simulink model "LSSB"  (R2013b)
settings: Solver=ode45  StartTime=0.0  StopTime=10.0  RelTol=1e-3
undefined symbols (not defined in the file): fdesignblkfcn, gcbh
libraries: dspsrcs4 x1
settings Model: Creator=Nouri  LastModifiedBy=Nouri

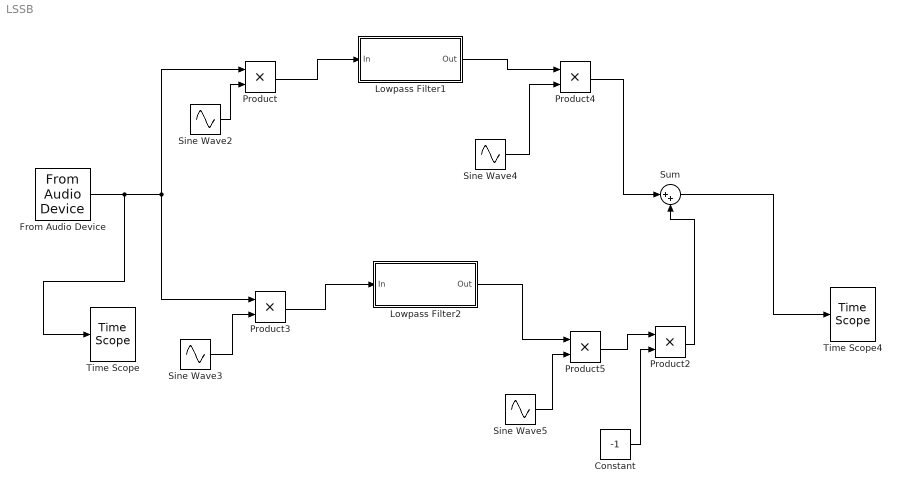
== system LSSB ==
  Constant : Constant  Value=-1
  From Audio Device : dspsrcs4/From Audio Device  deviceName=Default  numChannels=1  sampleRate=44000  deviceDatatype=Determine from output data type  autoBufferSize=on  bufferSize=4096  queueDuration=5  frameSize=1  outputDatatype=single  defaultInputChannelMapping=on  inputChannelMapping=1:2
  Lowpass Filter1 : Subsystem  DialogController=fdesignblkfcn  InitFcn=fdesignblkfcn(gcbh, {'InitFcn'});  mask(Lowpass Filter){}
      mask help: Design a lowpass filter
      settings: CopyFcn=fdesignblkfcn(gcbh, {'CopyFcn'});
      mask Help: helpview(mapfilelocation('dsp'), 'dsplowpassfilter');
      mask Display: disp('Lowpass')
  Lowpass Filter2 : Subsystem  DialogController=fdesignblkfcn  InitFcn=fdesignblkfcn(gcbh, {'InitFcn'});  mask(Lowpass Filter){}
      mask help: Design a lowpass filter
      settings: CopyFcn=fdesignblkfcn(gcbh, {'CopyFcn'});
      mask Help: helpview(mapfilelocation('dsp'), 'dsplowpassfilter');
      mask Display: disp('Lowpass')
  Product{,2..5} (5 alike) : Product
  Sine Wave2 : Sin  Amplitude=5  Frequency=22000  Phase=pi/2  SampleTime=0
  Sine Wave3 : Sin  Amplitude=5  Frequency=22000  SampleTime=0
  Sine Wave4 : Sin  Amplitude=5  Frequency=66000  Phase=pi/2  SampleTime=0
  Sine Wave5 : Sin  Amplitude=5  Frequency=66000  SampleTime=0
  Sum : Sum  Inputs=|++
  Time Scope : TimeScope  DefaultConfigurationName=spbscopes.TimeScopeBlockCfg
      settings: CopyFcn=scopeextensions.ScopeBlock.onCoreBlockCopy(gcbh);  DeleteFcn=scopeextensions.ScopeBlock.callback(gcbh, 'onBlockDelete');  PreSaveFcn=scopeextensions.ScopeBlock.callback(gcbh, 'onModelSave');  NameChangeFcn=scopeextensions.ScopeBlock.callback(gcbh, 'onBlockRename');  DestroyFcn=scopeextensions.ScopeBlock.onBlockDestroy(gcbh)  CloseFcn=scopeextensions.ScopeBlock.callback(gcbh, 'onBlockClose');  PreDeleteFcn=scopeextensions.ScopeBlock.callback(gcbh, 'onBlockPreDelete');
  Time Scope4 : TimeScope  DefaultConfigurationName=spbscopes.TimeScopeBlockCfg
      settings: CopyFcn=scopeextensions.ScopeBlock.onCoreBlockCopy(gcbh);  DeleteFcn=scopeextensions.ScopeBlock.callback(gcbh, 'onBlockDelete');  PreSaveFcn=scopeextensions.ScopeBlock.callback(gcbh, 'onModelSave');  NameChangeFcn=scopeextensions.ScopeBlock.callback(gcbh, 'onBlockRename');  DestroyFcn=scopeextensions.ScopeBlock.onBlockDestroy(gcbh)  CloseFcn=scopeextensions.ScopeBlock.callback(gcbh, 'onBlockClose');  PreDeleteFcn=scopeextensions.ScopeBlock.callback(gcbh, 'onBlockPreDelete');
  wires:
  Sine Wave2/1 -> Product/2
  From Audio Device/1 -> Product/1, Product3/1, Time Scope/1
  Sine Wave3/1 -> Product3/2
  Product/1 -> Lowpass Filter1/1(In)
  Product3/1 -> Lowpass Filter2/1(In)
  Lowpass Filter2/1(Out) -> Product5/1
  Lowpass Filter1/1(Out) -> Product4/1
  Sine Wave4/1 -> Product4/2
  Sine Wave5/1 -> Product5/2
  Product4/1 -> Sum/1
  Sum/1 -> Time Scope4/1
  Product5/1 -> Product2/1
  Constant/1 -> Product2/2
  Product2/1 -> Sum/2

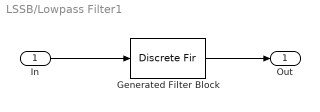
== system LSSB/Lowpass Filter1 ==
  In : Inport
  Generated Filter Block : DiscreteFir  Tag=BlockMethodSubSystem  Coefficients=[-0.0034436495845580231 -0.0059164791571934081 0.0074434606687912869 0.054740018373940491 0.13478679515848707 0.21479383660135923 0.24873045448052369 0.21479383660135923 0.13478679515848707 0.054740018373940491 0.0074434606687912869 -0.0059164791571934081 -0.0034436495845580231]
  Out : Outport
  wires:
  In/1 -> Generated Filter Block/1
  Generated Filter Block/1 -> Out/1

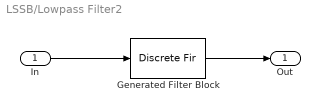
== system LSSB/Lowpass Filter2 ==
  In : Inport
  Generated Filter Block : DiscreteFir  Tag=BlockMethodSubSystem  Coefficients=[-0.0034436495845580231 -0.0059164791571934081 0.0074434606687912869 0.054740018373940491 0.13478679515848707 0.21479383660135923 0.24873045448052369 0.21479383660135923 0.13478679515848707 0.054740018373940491 0.0074434606687912869 -0.0059164791571934081 -0.0034436495845580231]
  Out : Outport
  wires:
  In/1 -> Generated Filter Block/1
  Generated Filter Block/1 -> Out/1
